simulink model "observer_dynami"  (R2018b)
settings: Solver=VariableStepAuto  StartTime=0.0  StopTime=10.0  RelTol=1e-3
values from neighbouring files (symbols this model uses):
  A = double(A)    [Linearization.m]    (also in findK_emtiazi.m = [1 2 0; 0 -1 3; 0 1 -1])
  B = double(B)    [Linearization.m]
  C = [1 0 0 0 ; 0 1 0 0 ]    [Linearization.m]    (also in findK_emtiazi.m = [0 1 0])
  k = place(A,B,pc)    [Linearization.m]
  l = place(A',C',po)'    [Linearization.m]    (also in findK_emtiazi.m = rank(Wc))
settings Model: Creator=sepehr  LastModifiedBy=sepehr

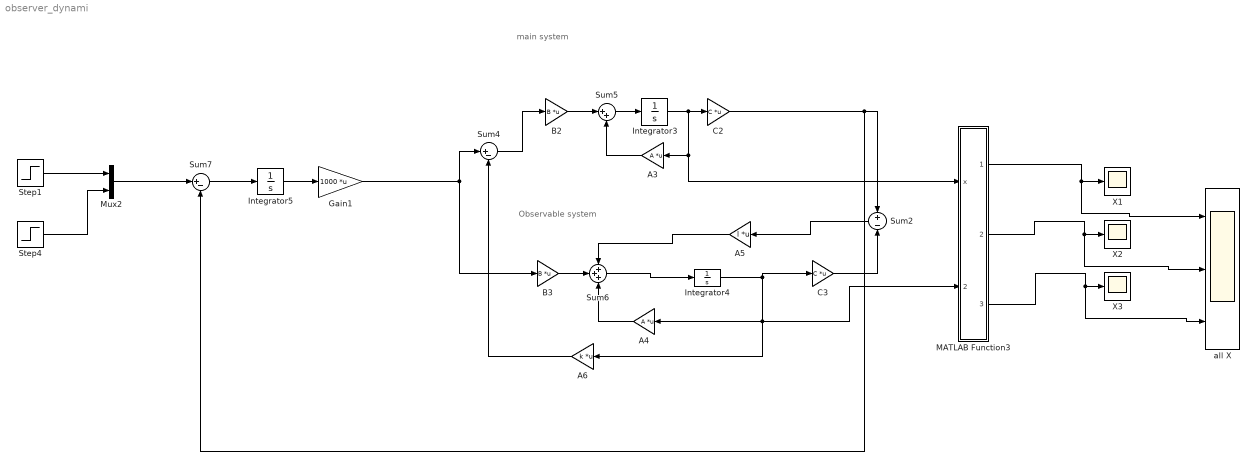
== system observer_dynami ==
  note: main system
  note: Observable system
  A3 : Gain  Gain=A  Multiplication=Matrix(K*u) (u vector)
  A4 : Gain  Gain=A  Multiplication=Matrix(K*u) (u vector)
  A5 : Gain  Gain=l  Multiplication=Matrix(K*u) (u vector)
  A6 : Gain  Gain=k  Multiplication=Matrix(K*u) (u vector)
  B2 : Gain  Gain=B  Multiplication=Matrix(K*u) (u vector)
  B3 : Gain  Gain=B  Multiplication=Matrix(K*u) (u vector)
  C2 : Gain  Gain=C  Multiplication=Matrix(K*u) (u vector)
  C3 : Gain  Gain=C  Multiplication=Matrix(K*u) (u vector)
  Gain1 : Gain  Gain=1000  Multiplication=Matrix(K*u)
  Integrator3 : Integrator
  Integrator4 : Integrator
  Integrator5 : Integrator  InitialCondition=0.5
  MATLAB Function3 : MATLAB Function  TreatAsAtomicUnit=on
  Mux2 : Mux  Inputs=2
  Step1 : Step  Time=0  SampleTime=0.0001
  Step4 : Step  Time=0  After=1.2  SampleTime=0.001
  Sum2 : Sum  Inputs=+-
  Sum4 : Sum  Inputs=|+-
  Sum5 : Sum  Inputs=|++
  Sum6 : Sum  Inputs=+++
  Sum7 : Sum  Inputs=|+-
  X1 : Scope
  X2 : Scope
  X3 : Scope
  all X : Scope  NumInputPorts=3
  wires:
  Sum4/1 -> B2/1
  Step1/1 -> Mux2/1
  Integrator3/1 -> A3/1, MATLAB Function3/1(x), C2/1
  B3/1 -> Sum6/2
  B2/1 -> Sum5/1
  C3/1 -> Sum2/2
  A4/1 -> Sum6/3
  C2/1 -> Sum2/1, Sum7/2
  Sum2/1 -> A5/1
  MATLAB Function3/2(x2) -> all X/2, X2/1
  MATLAB Function3/3(x3) -> all X/3, X3/1
  Sum5/1 -> Integrator3/1
  Integrator4/1 -> C3/1, A6/1, A4/1, MATLAB Function3/2(x_hat)
  A5/1 -> Sum6/1
  A6/1 -> Sum4/2
  A3/1 -> Sum5/2
  MATLAB Function3/1(x1) -> all X/1, X1/1
  Step4/1 -> Mux2/2
  Sum6/1 -> Integrator4/1
  Integrator5/1 -> Gain1/1
  Gain1/1 -> Sum4/1, B3/1
  Sum7/1 -> Integrator5/1
  Mux2/1 -> Sum7/1

== matlab function observer_dynami/MATLAB Function3 ==
  data: x input; x_hat input; x1 output; x2 output; x3 output
function [x1,x2,x3] = CP(x,x_hat)

x1=[x(1),x_hat(1)];
x2=[x(2),x_hat(2)];
x3=[x(3),x_hat(3)];
